simulink model "test_stability_link_neuron_sense_all"  (R2022a)
settings: Solver=VariableStepAuto  StartTime=0.0  StopTime=20.0  RelTol=1e-3
values from neighbouring files (symbols this model uses):
  Y = fft(theta)    [testStability.m]    (also in testStabilityTmp2.m)
undefined symbols (not defined in the file or in its folder): dfm, dfm_s, dsm, dsm_s, dsp, dsp_s, dsyn_s, dup, dup_s, gfm, gfm_s, gsm, gsm_s, gsp, gsp_s, gsyn_s, gup, gup_s, Iapp, Iapp_s, max_torque, noisePwr, rflx_g, sampleTime, X, Z
libraries: sm_lib x6, nesl_utility x4, simulink x2
settings Model: Creator=chris  LastModifiedBy=chris

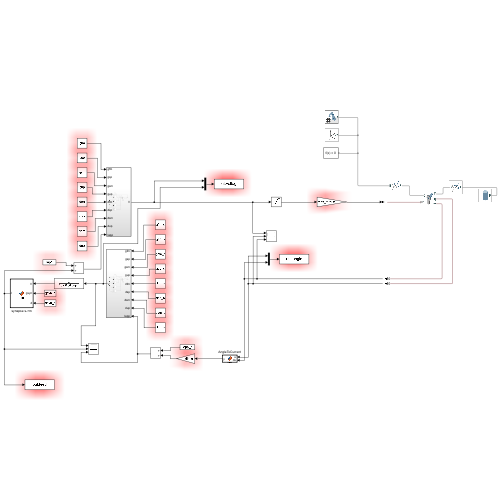
[thumbnail: Simulink's stored preview of the top-level diagram]
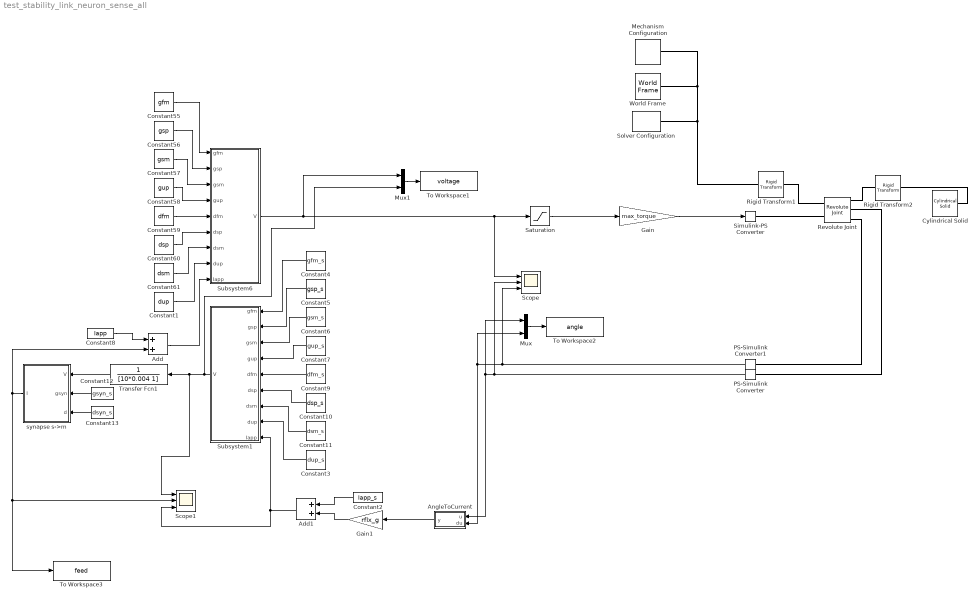
== system test_stability_link_neuron_sense_all ==
  Add : Sum
  Add1 : Sum
  AngleToCurrent : MATLAB Function  TreatAsAtomicUnit=on
  Constant1 : Constant  Value=dup
  Constant10 : Constant  Value=dsp_s
  Constant11 : Constant  Value=dsm_s
  Constant12 : Constant  Value=gsyn_s
  Constant13 : Constant  Value=dsyn_s
  Constant2 : Constant  Value=Iapp_s
  Constant3 : Constant  Value=dup_s
  Constant4 : Constant  Value=gfm_s
  Constant5 : Constant  Value=gsp_s
  Constant55 : Constant  Value=gfm
  Constant56 : Constant  Value=gsp
  Constant57 : Constant  Value=gsm
  Constant58 : Constant  Value=gup
  Constant59 : Constant  Value=dfm
  Constant6 : Constant  Value=gsm_s
  Constant60 : Constant  Value=dsp
  Constant61 : Constant  Value=dsm
  Constant7 : Constant  Value=gup_s
  Constant8 : Constant  Value=Iapp
  Constant9 : Constant  Value=dfm_s
  Cylindrical Solid : sm_lib/Body Elements/Cylindrical Solid  GraphicAmbientColor=[0.15 0.15 0.15 1.0]  BasedOnType=Density  CenterOfMass=[0 0 0]  CenterOfMassUnits=m  GraphicDiffuseColor=[0.5 0.5 0.5]  CylinderLength=0.5  CylinderLengthUnits=m  CylinderRadius=0.05  CylinderRadiusUnits=m  Density=1000  DensityUnits=kg/m^3  DoExposeReferenceFrame=on  GraphicEmissiveColor=[0.0 0.0 0.0 1.0]  ExportEntireGeometry=off  SerializedFrames=<Frames/>  MarkerShape=Sphere  MarkerSize=10  GraphicType=FromGeometry  InertiaType=CalculateFromGeometry  Mass=1  MassUnits=kg  MomentsOfInertia=[1 1 1]  MomentsOfInertiaUnits=kg*m^2  GraphicOpacity=1.0  ProductsOfInertia=[0 0 0]  ProductsOfInertiaUnits=kg*m^2  GraphicShininess=75  GraphicSpecularColor=[0.5 0.5 0.5 1.0]  GraphicVisPropType=SimpleVisualProperties
  Gain : Gain  Gain=max_torque
  Gain1 : Gain  Gain=rflx_g
  Mechanism Configuration : sm_lib/Utilities/Mechanism Configuration  UniformGravity=Constant  GravityVector=[0 0 -9.80665]  GravityUnits=m/s^2  LinearizationDelta=0.001  JointModeTransitionNonlinearIterations=2
  Mux : Mux  Inputs=2
  Mux1 : Mux  Inputs=2
  PS-Simulink Converter : nesl_utility/PS-Simulink Converter  PhysicalDomain=network_engine_domain  SubClassName=ps_output  LeftPortType=input  RightPortType=output  PseudoPeriodic=off  Frequencies=[]  VectorFormat=inherit  Unit=inherit  AffineConversion=off
      settings: SourceProductBaseCode=SS,PW,VE
  PS-Simulink Converter1 : nesl_utility/PS-Simulink Converter  PhysicalDomain=network_engine_domain  SubClassName=ps_output  LeftPortType=input  RightPortType=output  PseudoPeriodic=off  Frequencies=[]  VectorFormat=inherit  Unit=inherit  AffineConversion=off
      settings: SourceProductBaseCode=SS,PW,VE
  Revolute Joint : sm_lib/Joints/Revolute Joint  JointMode=Normal  SenseConstraintForce=off  SenseConstraintForceX=off  SenseConstraintForceY=off  SenseConstraintForceZ=off  SenseConstraintTorque=off  SenseConstraintTorqueX=off  SenseConstraintTorqueY=off  SenseConstraintTorqueZ=off  SenseTotalForce=off  SenseTotalForceX=off  SenseTotalForceY=off  SenseTotalForceZ=off  SenseTotalTorque=off  SenseTotalTorqueX=off  SenseTotalTorqueY=off  SenseTotalTorqueZ=off  CompositeWrenchDir=FollowerOnBase  CompositeWrenchFrame=BaseFrame  EquilibriumPosition=0  EquilibriumPositionUnits=deg  SpringStiffness=0.0  SpringStiffnessUnits=N*m/deg  DampingCoefficient=0.01  DampingCoefficientUnits=N*m*s/deg  TorqueActuationMode=InputTorque  MotionActuationMode=ComputedMotion  SensePosition=on  SenseVelocity=on  SenseAcceleration=off  SenseTorqueForce=off  SenseLowerLimitTorqueForce=off  SenseUpperLimitTorqueForce=off  LowerLimitSpecify=off  LowerLimitBound=-90  LowerLimitBoundUnits=deg  LowerLimitStiffness=1e4  LowerLimitStiffnessUnits=N*m/deg  LowerLimitDamping=10  LowerLimitDampingUnits=N*m/(deg/s)  LowerLimitTransitionRegionWidth=0.1  LowerLimitTransitionRegionWidthUnits=deg  UpperLimitSpecify=off  UpperLimitBound=90  UpperLimitBoundUnits=deg  UpperLimitStiffness=1e4  UpperLimitStiffnessUnits=N*m/deg  UpperLimitDamping=10  UpperLimitDampingUnits=N*m/(deg/s)  UpperLimitTransitionRegionWidth=0.1  UpperLimitTransitionRegionWidthUnits=deg  PositionTargetSpecify=on  PositionTargetPriority=High  PositionTargetValue=20  PositionTargetValueUnits=deg  VelocityTargetSpecify=off  VelocityTargetPriority=High  VelocityTargetValue=0  VelocityTargetValueUnits=deg/s
  Rigid Transform1 : sm_lib/Frames and Transforms/Rigid Transform  TranslationMethod=None  TranslationStandardOffset=0.25  TranslationLengthUnit=m  TranslationStandardAxis=+X  TranslationCartesianOffset=[0 0 0]  TranslationROffset=0  TranslationROffsetUnits=m  TranslationZOffset=0  TranslationZOffsetUnits=m  TranslationThetaOffset=0  TranslationThetaOffsetUnits=deg  RotationMethod=RotationSequence  RotationAngleUnits=deg  RotationStandardAxis=+Y  RotationAngle=90  RotationArbitraryAxis=[0 0 1]  FollAlignAxisA=+X  BaseAlignAxisA=+Y  FollAlignAxisB=+Y  BaseAlignAxisB=+Z  RotationSequenceAxes=FollowerAxes  RotationSequence=XYX  RotationSequenceAngles=[0 90 90]  RotationSequenceAnglesUnits=deg  RotationMatrix=[1 0 0; 0 1 0; 0 0 1]
  Rigid Transform2 : sm_lib/Frames and Transforms/Rigid Transform  TranslationMethod=StandardAxis  TranslationStandardOffset=.25  TranslationLengthUnit=m  TranslationStandardAxis=+X  TranslationCartesianOffset=[0 0 0]  TranslationROffset=0  TranslationROffsetUnits=m  TranslationZOffset=0  TranslationZOffsetUnits=m  TranslationThetaOffset=0  TranslationThetaOffsetUnits=deg  RotationMethod=RotationSequence  RotationAngleUnits=deg  RotationStandardAxis=+Z  RotationAngle=90  RotationArbitraryAxis=[0 0 1]  FollAlignAxisA=+X  BaseAlignAxisA=+Y  FollAlignAxisB=+Y  BaseAlignAxisB=+Z  RotationSequenceAxes=FollowerAxes  RotationSequence=XYX  RotationSequenceAngles=[0 90 0]  RotationSequenceAnglesUnits=deg  RotationMatrix=[1 0 0; 0 1 0; 0 0 1]
  Saturation : Saturate  UpperLimit=1.0  LowerLimit=0.0
  Scope : Scope  NumInputPorts=3
  Scope1 : Scope  NumInputPorts=3
  Simulink-PS Converter : nesl_utility/Simulink-PS Converter  PhysicalDomain=network_engine_domain  SubClassName=ps_input  LeftPortType=input  RightPortType=output  PseudoPeriodic=off  Frequencies=[]  NoiseDistribution=none  NoiseParameters=[]  Unit=1  AffineConversion=off  FilteringAndDerivatives=provide  SimscapeFilterOrder=1  InputFilterTimeConstant=0.001  UdotUserProvided=0
      settings: SourceProductBaseCode=SS,PW,VE
  Solver Configuration : nesl_utility/Solver Configuration  PhysicalDomain=network_engine_domain  SubClassName=solver  LeftPortType=input  RightPortType=generic  Tones=[]  Harmonics=[]  SimulateNoise=off  Profile=off  UseLocalSampling=off  EnableSwitchedLinearOptims=on  FrequencyDomain=off  UseCCode=off  RelTol=0.001  AbsTol=1e-06  MinStep=1e-09  ToWorkspace=off  RevertToSquareIcSolve=off  NumHomotopyIterations=100  PhasorMode=off  PhasorModeNumHarmonics=1  IndexReductionMethod=DerivativeReplacement  DoDC=off  ResidualTolerance=1e-09  UseLocalSolver=off  LocalSolverChoice=NE_BACKWARD_EULER_ADVANCER  LocalSolverSampleTime=0.001  DoFixedCost=off  MaxNonlinIter=3  MaxModeIter=2  ComputeImpulses=off  ImpulseIterations=2  LinearAlgebra=auto  LinearAlgebraNumThread=0  EquationFormulation=NE_TIME_EF  DelaysMemoryBudget=1024  AutomaticFiltering=on  FilteringTimeConstant=0.001  PartitionStorageMethod=AS_NEEDED  PartitionMemoryBudget=1024  PartitionMethod=ROBUST
      settings: SourceProductBaseCode=SS,PW,VE
  Subsystem1 : Subsystem
  Subsystem6 : Subsystem
  To Workspace1 : ToWorkspace  VariableName=voltage  SaveFormat=Structure With Time  SampleTime=sampleTime
  To Workspace2 : ToWorkspace  VariableName=angle  SaveFormat=Structure With Time  SampleTime=sampleTime
  To Workspace3 : ToWorkspace  VariableName=feed  SaveFormat=Structure With Time  SampleTime=sampleTime
  Transfer Fcn1 : TransferFcn  Denominator=[10*0.004 1]
  World Frame : sm_lib/Frames and Transforms/World Frame
  synapse s->m : MATLAB Function  TreatAsAtomicUnit=on
  wires:
  Subsystem6/1(V) -> Mux1/1, Scope/1, Saturation/1
  Constant60/1 -> Subsystem6/6(dsp)
  Constant1/1 -> Subsystem6/8(dup)
  Constant59/1 -> Subsystem6/5(dfm)
  Constant57/1 -> Subsystem6/3(gsm)
  Constant61/1 -> Subsystem6/7(dsm)
  Constant56/1 -> Subsystem6/2(gsp)
  Constant58/1 -> Subsystem6/4(gup)
  Constant55/1 -> Subsystem6/1(gfm)
  Saturation/1 -> Gain/1
  Add/1 -> Subsystem6/9(Iapp)
  Gain/1 -> Simulink-PS Converter/1
  PS-Simulink Converter/1 -> Mux/1, AngleToCurrent/1(u), Scope/2
  Constant8/1 -> Add/1
  Mux/1 -> To Workspace2/1
  PS-Simulink Converter1/1 -> Scope/3, Mux/2, AngleToCurrent/2(du)
  Constant2/1 -> Add1/1
  Gain1/1 -> Add1/2
  Add1/1 -> Scope1/3, Subsystem1/9(Iapp)
  AngleToCurrent/1(y) -> Gain1/1
  Constant7/1 -> Subsystem1/4(gup)
  Constant9/1 -> Subsystem1/5(dfm)
  Constant5/1 -> Subsystem1/2(gsp)
  Constant4/1 -> Subsystem1/1(gfm)
  Constant10/1 -> Subsystem1/6(dsp)
  Constant6/1 -> Subsystem1/3(gsm)
  Constant3/1 -> Subsystem1/8(dup)
  Constant11/1 -> Subsystem1/7(dsm)
  Constant12/1 -> synapse s->m/2(gsyn)
  Constant13/1 -> synapse s->m/3(d)
  Subsystem1/1(V) -> Mux1/2, Scope1/1, Transfer Fcn1/1
  Transfer Fcn1/1 -> synapse s->m/1(V)
  Mux1/1 -> To Workspace1/1
  synapse s->m/1(I) -> Add/2, To Workspace3/1, Scope1/2
  connections:
  Solver Configuration/RConn1 -- Mechanism Configuration/RConn1 -- World Frame/RConn1 -- Rigid Transform1/LConn1
  Rigid Transform1/RConn1 -- Revolute Joint/LConn1
  Simulink-PS Converter/RConn1 -- Revolute Joint/LConn2
  Rigid Transform2/RConn1 -- Cylindrical Solid/RConn1
  Rigid Transform2/LConn1 -- Revolute Joint/RConn1
  Revolute Joint/RConn2 -- PS-Simulink Converter/LConn1
  PS-Simulink Converter1/LConn1 -- Revolute Joint/RConn3

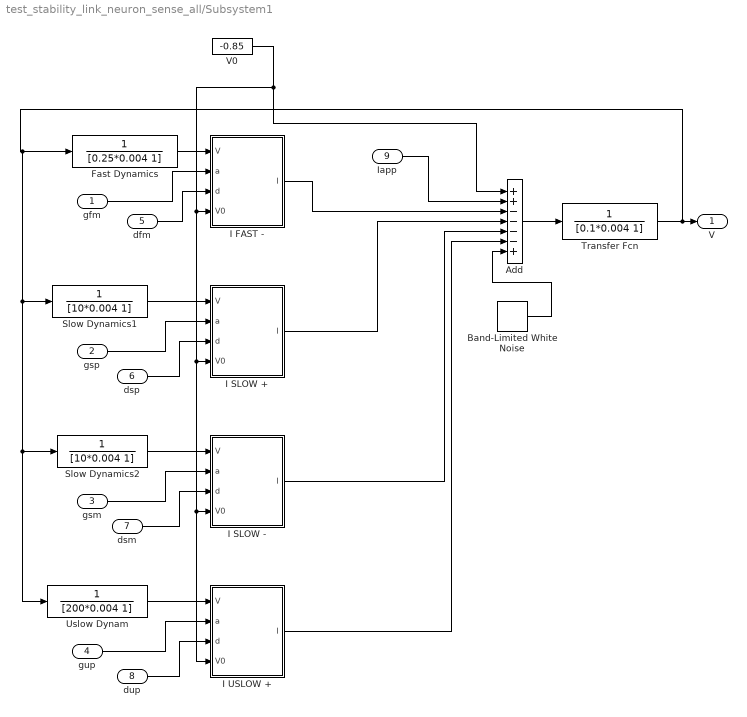
== system test_stability_link_neuron_sense_all/Subsystem1 ==
  gfm : Inport
  gsp : Inport  Port=2
  gsm : Inport  Port=3
  gup : Inport  Port=4
  dfm : Inport  Port=5
  dsp : Inport  Port=6
  dsm : Inport  Port=7
  dup : Inport  Port=8
  Iapp : Inport  Port=9
  Add : Sum  Inputs=++----+
  Band-Limited White Noise : simulink/Sources/Band-Limited White Noise  Cov=[noisePwr]  Ts=0.001  seed=floor(rand(1)*250000)
  Fast Dynamics : TransferFcn  Denominator=[0.25*0.004 1]
  I FAST - : MATLAB Function  TreatAsAtomicUnit=on
  I SLOW + : MATLAB Function  TreatAsAtomicUnit=on
  I SLOW - : MATLAB Function  TreatAsAtomicUnit=on
  I USLOW + : MATLAB Function  TreatAsAtomicUnit=on
  Slow Dynamics1 : TransferFcn  Denominator=[10*0.004 1]
  Slow Dynamics2 : TransferFcn  Denominator=[10*0.004 1]
  Transfer Fcn : TransferFcn  Denominator=[0.1*0.004 1]
  Uslow Dynam : TransferFcn  Denominator=[200*0.004 1]
  V0 : Constant  Value=-0.85
  V : Outport
  wires:
  dup/1 -> I USLOW +/3(d)
  gsm/1 -> I SLOW -/2(a)
  dsm/1 -> I SLOW -/3(d)
  gup/1 -> I USLOW +/2(a)
  Iapp/1 -> Add/2
  Uslow Dynam/1 -> I USLOW +/1(V)
  Add/1 -> Transfer Fcn/1
  Slow Dynamics1/1 -> I SLOW +/1(V)
  Slow Dynamics2/1 -> I SLOW -/1(V)
  I FAST -/1(I) -> Add/3
  I USLOW +/1(I) -> Add/6
  V0/1 -> I USLOW +/4(V0), I SLOW -/4(V0), I SLOW +/4(V0), I FAST -/4(V0), Add/1
  dsp/1 -> I SLOW +/3(d)
  gsp/1 -> I SLOW +/2(a)
  dfm/1 -> I FAST -/3(d)
  gfm/1 -> I FAST -/2(a)
  Fast Dynamics/1 -> I FAST -/1(V)
  I SLOW -/1(I) -> Add/5
  Transfer Fcn/1 -> Uslow Dynam/1, Slow Dynamics2/1, Slow Dynamics1/1, Fast Dynamics/1, V/1
  I SLOW +/1(I) -> Add/4
  Band-Limited White Noise/1 -> Add/7

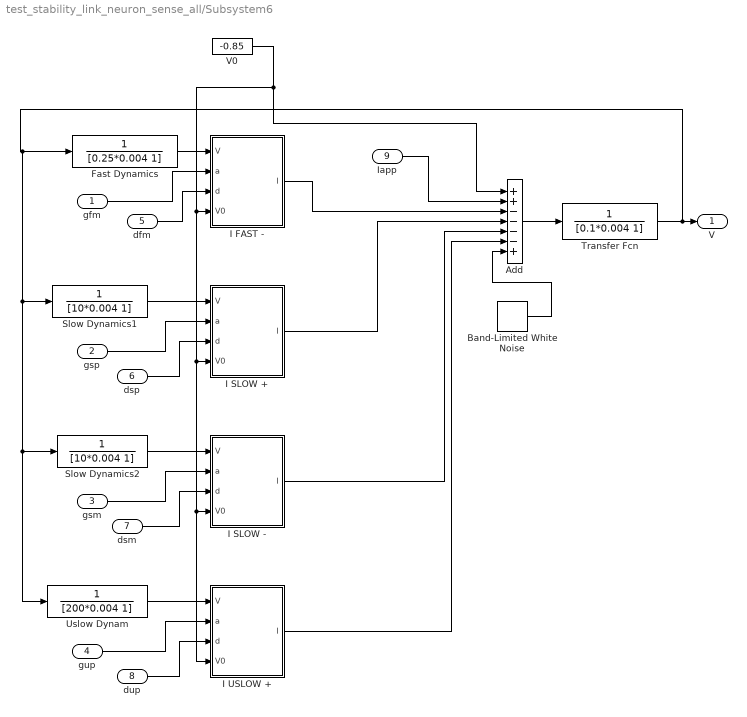
== system test_stability_link_neuron_sense_all/Subsystem6 ==
  gfm : Inport
  gsp : Inport  Port=2
  gsm : Inport  Port=3
  gup : Inport  Port=4
  dfm : Inport  Port=5
  dsp : Inport  Port=6
  dsm : Inport  Port=7
  dup : Inport  Port=8
  Iapp : Inport  Port=9
  Add : Sum  Inputs=++----+
  Band-Limited White Noise : simulink/Sources/Band-Limited White Noise  Cov=[noisePwr]  Ts=0.001  seed=floor(rand(1)*250000)
  Fast Dynamics : TransferFcn  Denominator=[0.25*0.004 1]
  I FAST - : MATLAB Function  TreatAsAtomicUnit=on
  I SLOW + : MATLAB Function  TreatAsAtomicUnit=on
  I SLOW - : MATLAB Function  TreatAsAtomicUnit=on
  I USLOW + : MATLAB Function  TreatAsAtomicUnit=on
  Slow Dynamics1 : TransferFcn  Denominator=[10*0.004 1]
  Slow Dynamics2 : TransferFcn  Denominator=[10*0.004 1]
  Transfer Fcn : TransferFcn  Denominator=[0.1*0.004 1]
  Uslow Dynam : TransferFcn  Denominator=[200*0.004 1]
  V0 : Constant  Value=-0.85
  V : Outport
  wires:
  dup/1 -> I USLOW +/3(d)
  gsm/1 -> I SLOW -/2(a)
  dsm/1 -> I SLOW -/3(d)
  gup/1 -> I USLOW +/2(a)
  Iapp/1 -> Add/2
  Uslow Dynam/1 -> I USLOW +/1(V)
  Add/1 -> Transfer Fcn/1
  Slow Dynamics1/1 -> I SLOW +/1(V)
  Slow Dynamics2/1 -> I SLOW -/1(V)
  I FAST -/1(I) -> Add/3
  I USLOW +/1(I) -> Add/6
  V0/1 -> I USLOW +/4(V0), I SLOW -/4(V0), I SLOW +/4(V0), I FAST -/4(V0), Add/1
  dsp/1 -> I SLOW +/3(d)
  gsp/1 -> I SLOW +/2(a)
  dfm/1 -> I FAST -/3(d)
  gfm/1 -> I FAST -/2(a)
  Fast Dynamics/1 -> I FAST -/1(V)
  I SLOW -/1(I) -> Add/5
  Transfer Fcn/1 -> Uslow Dynam/1, Slow Dynamics2/1, Slow Dynamics1/1, Fast Dynamics/1, V/1
  I SLOW +/1(I) -> Add/4
  Band-Limited White Noise/1 -> Add/7

== matlab function test_stability_link_neuron_sense_all/Subsystem1/I FAST - ==
  data: V input; I output; a input; d input; V0 input
function I = fcn(V,a,d,V0)

I = a*(tanh(V-d)-tanh(V0-d));

== matlab function test_stability_link_neuron_sense_all/Subsystem1/I SLOW + ==
  data: V input; I output; a input; d input; V0 input
function I = fcn(V,a,d,V0)

I = a*(tanh(V-d)-tanh(V0-d));

== matlab function test_stability_link_neuron_sense_all/Subsystem1/I SLOW - ==
  data: V input; I output; a input; d input; V0 input
function I = fcn(V,a,d,V0)

I = a*(tanh(V-d)-tanh(V0-d));

== matlab function test_stability_link_neuron_sense_all/Subsystem1/I USLOW + ==
  data: V input; I output; a input; d input; V0 input
function I = fcn(V,a,d,V0)

I = a*(tanh(V-d)-tanh(V0-d));

== matlab function test_stability_link_neuron_sense_all/AngleToCurrent ==
  data: u input; y output; du input
function y = fcn(u, du)
%y = 0.5*(1+tanh(50*(u))) - 0.5*(-tanh(50*(u+0.3)) + 1);
%y = min(sign(u), u);
uy = (1-tanh(15*(sin(u)-0.05)))/2 -1 ;
duy = (tanh(5*(du+0.5)) - tanh(5*(du-0.5)))/2 - 1;
y = uy + duy;
%duy = 2-(tanh(5*(du+0.5)) - tanh(5*(du-0.5)));
%y = u-;

== matlab function test_stability_link_neuron_sense_all/synapse s->m ==
  data: V input; I output; gsyn input; d input
function I = fcn(V,gsyn,d)

I = gsyn*(tanh(2*(V-d))+1)/2;

== matlab function test_stability_link_neuron_sense_all/Subsystem6/I FAST - ==
  data: V input; I output; a input; d input; V0 input
function I = fcn(V,a,d,V0)

I = a*(tanh(V-d)-tanh(V0-d));

== matlab function test_stability_link_neuron_sense_all/Subsystem6/I SLOW + ==
  data: V input; I output; a input; d input; V0 input
function I = fcn(V,a,d,V0)

I = a*(tanh(V-d)-tanh(V0-d));

== matlab function test_stability_link_neuron_sense_all/Subsystem6/I SLOW - ==
  data: V input; I output; a input; d input; V0 input
function I = fcn(V,a,d,V0)

I = a*(tanh(V-d)-tanh(V0-d));

== matlab function test_stability_link_neuron_sense_all/Subsystem6/I USLOW + ==
  data: V input; I output; a input; d input; V0 input
function I = fcn(V,a,d,V0)

I = a*(tanh(V-d)-tanh(V0-d));
